simulink model "Simulink_B_8_4"  (R2017b)
settings: Solver=VariableStepAuto  StartTime=0.0  StopTime=10.0  RelTol=1e-3
settings Model: Creator=LUCIA  LastModifiedBy=LUCIA

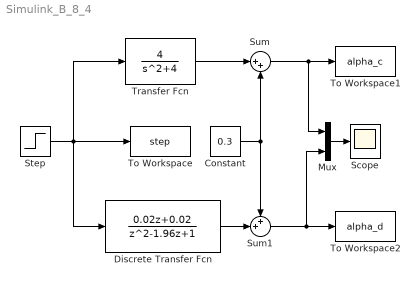
== system Simulink_B_8_4 ==
  Constant : Constant  Value=0.3
  Discrete Transfer Fcn : DiscreteTransferFcn  Numerator=[0.02 0.02]  Denominator=[1 -1.96 1]  SampleTime=0.1
  Mux : Mux  Inputs=2
  Scope : Scope
  Step : Step  After=8  SampleTime=0
  Sum : Sum  Inputs=|++
  Sum1 : Sum  Inputs=++|
  To Workspace : ToWorkspace  VariableName=step  SaveFormat=Timeseries  SampleTime=-1
  To Workspace1 : ToWorkspace  VariableName=alpha_c  SaveFormat=Timeseries  SampleTime=-1
  To Workspace2 : ToWorkspace  VariableName=alpha_d  SaveFormat=Timeseries  SampleTime=-1
  Transfer Fcn : TransferFcn  Numerator=4  Denominator=[1 0 4]
  wires:
  Transfer Fcn/1 -> Sum/1
  Constant/1 -> Sum1/1, Sum/2
  Discrete Transfer Fcn/1 -> Sum1/2
  Step/1 -> To Workspace/1, Discrete Transfer Fcn/1, Transfer Fcn/1
  Sum/1 -> To Workspace1/1, Mux/1
  Sum1/1 -> To Workspace2/1, Mux/2
  Mux/1 -> Scope/1
